simulink model "SS_controller_v01"  (R2019a)
settings: Solver=VariableStepAuto  StartTime=0.0  StopTime=10.0  RelTol=1e-3
values from neighbouring files (symbols this model uses):
  A = [ deriv.x_u,    deriv.x_w,	deriv.x_q,	deriv.x_theta,  0 ... (first row only)    [control_system_v01.m]    (also in control_system_v02.m = [ deriv.x_u,    deriv.x_w,	deriv.x_q,	deriv.x_theta)
  B = [   deriv.x_eta,    deriv.x_tau ... (first row only)    [control_system_v01.m]    (also in control_system_v02.m)
  C = [0 0 1 0 0]    [control_system_v01.m]    (also in control_system_v02.m = eye(4))
  D = 0    [control_system_v01.m]    (also in control_system_v02.m = zeros(size(C,1),size(B,2)))
settings Model: Creator=tyson  LastModifiedBy=tyson

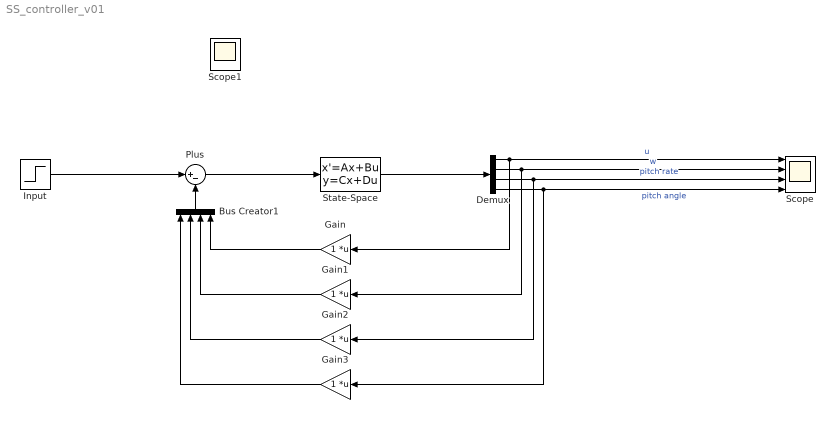
== system SS_controller_v01 ==
  Bus Creator1 : BusCreator  Inputs=4
  Demux : Demux
  Gain{,1..3} (4 alike) : Gain  Multiplication=Matrix(K*u)
  Input : Step
  Plus : Sum  Inputs=|+-
  Scope : Scope  NumInputPorts=4
  State-Space : StateSpace  A=A  B=B  C=C  D=D  InitialCondition=0
  Scope1 : Scope
  wires:
  Input/1 -> Plus/1
  Plus/1 -> State-Space/1
  State-Space/1 -> Demux/1
  Demux/1 -> Gain/1, Scope/1  "u"
  Demux/2 -> Gain1/1, Scope/2  "w"
  Demux/3 -> Gain2/1, Scope/3  "pitch rate"
  Demux/4 -> Gain3/1, Scope/4  "pitch angle"
  Bus Creator1/1 -> Plus/2
  Gain/1 -> Bus Creator1/4
  Gain1/1 -> Bus Creator1/3
  Gain2/1 -> Bus Creator1/2
  Gain3/1 -> Bus Creator1/1
